simulink model "QCar"  (R2018a)
settings: Solver=ode23t  StartTime=0.0  StopTime=10  EnableMultiTasking=on
PreLoadFcn:
  | load carParams
values from neighbouring files (symbols this model uses):
  b1 = 25    [matlab2.mat]
  b2 = 0    [matlab2.mat]
  k1 = 8100    [matlab2.mat]
  k2 = 23000    [matlab2.mat]
  mCar = 250    [matlab2.mat]
  mWheel = 60    [matlab2.mat]
settings Model: Creator=scastro  LastModifiedBy=Prana
settings DataIOCC: SaveFormat=Array  OutputTimes=0:0.001:60
settings OptimizationCC: LifeSpan=inf
settings DebuggingCC: SFUnexpectedBacktrackingDiag=warning  SFNoUnconditionalDefaultTransitionDiag=warning  SFExecutionAtInitializationDiag=none
settings HardwareCC: ProdBitPerPointer=32  ProdBitPerSizeT=32  ProdBitPerPtrDiffT=32  ProdLargestAtomicFloat=None  ProdIntDivRoundTo=Undefined  ProdEndianess=Unspecified  ProdWordSize=32  ProdHWDeviceType=32-bit Generic
settings ModelReferenceCC: PropagateSignalLabelsOutOfModel=off
settings CodeAppCC: StateflowObjectComments=on
settings GRTTargetCC: TargetLangStandard=C89/C90 (ANSI)  GeneratePreprocessorConditionals=Disable all
settings ConfigComp: CovMetricSettings=dw  CovHtmlReporting=on  CovSaveCumulativeToWorkspaceVar=on  CovSaveSingleToWorkspaceVar=on  CovExternalEMLEnable=off
settings SimscapeCC: SimscapeNormalizeSystem=off  SimscapeLogType=all  SimscapeLogDataHistory=10000
settings ConfigurationSet: Description=SimMechanics 2G

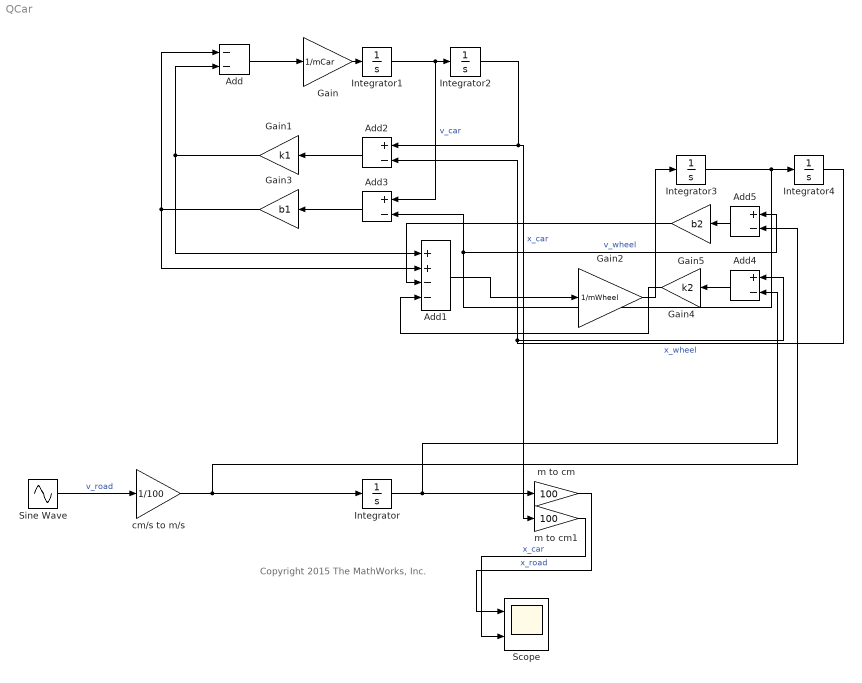
== system QCar ==
  note: Copyright 2015 The MathWorks, Inc.
  Add : Sum  Inputs=--
  Add1 : Sum  Inputs=++--
  Add{2..5} (4 alike) : Sum  Inputs=+-
  Gain : Gain  Gain=1/mCar
  Gain1 : Gain  Gain=k1
  Gain2 : Gain  Gain=1/mWheel
  Gain3 : Gain  Gain=b1
  Gain4 : Gain  Gain=k2
  Gain5 : Gain  Gain=b2
  Integrator{,1..4} (5 alike) : Integrator
  Scope : Scope  NumInputPorts=2
  Sine Wave : Sin  Amplitude=650  Frequency=100  Phase=pi/2  SampleTime=0
  cm/s to m/s : Gain  Gain=1/100
  m to cm : Gain  Gain=100
  m to cm1 : Gain  Gain=100
  wires:
  Integrator/1 -> Add4/2, m to cm/1
  cm/s to m/s/1 -> Add5/2, Integrator/1
  Gain/1 -> Integrator1/1
  Add/1 -> Gain/1
  Integrator2/1 -> Add2/1, m to cm1/1  "x_car"
  Integrator1/1 -> Add3/1, Integrator2/1  "v_car"
  Gain2/1 -> Integrator3/1
  Add1/1 -> Gain2/1
  Integrator4/1 -> Add2/2, Add4/1  "x_wheel"
  Integrator3/1 -> Add3/2, Add5/1, Integrator4/1  "v_wheel"
  Add2/1 -> Gain1/1
  Add3/1 -> Gain3/1
  Gain1/1 -> Add1/1, Add/2
  Gain3/1 -> Add1/2, Add/1
  Add4/1 -> Gain4/1
  Gain4/1 -> Add1/4
  Add5/1 -> Gain5/1
  Gain5/1 -> Add1/3
  Sine Wave/1 -> cm/s to m/s/1  "v_road"
  m to cm/1 -> Scope/1  "x_road"
  m to cm1/1 -> Scope/2  "x_car"
